simulink library "motdrv_lib"  (Simulink 7.5)
settings: Solver=ode45  StartTime=0.0  StopTime=10.0  RelTol=1e-3
settings Model: Creator=dauger  LastModifiedBy=dauger

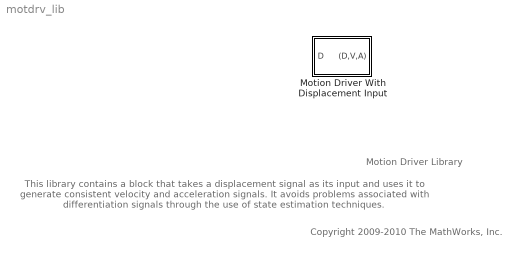
== system motdrv_lib ==
  note: Motion Driver Library
  note: This library contains a block that takes a displacement signal as its input and
      | uses it to generate consistent velocity and acceleration signals.  It avoids problems
      | associated with differentiation signals through the use of state estimation techniques.
  note: Copyright 2009-2010 The MathWorks, Inc.
  Motion Driver With Displacement Input : Subsystem  mask(Motion Driver with Acceleration Input){InitialDisplacement=0, InitialVelocity=0, TimeConstant=1}
      mask prompts: InitialDisplacement "Initial Displacement (units):"; InitialVelocity "Initial Velocity (units/s):"; TimeConstant "Time Constant (s):"
      mask help: This block takes as its input an acceleration and produces a three-dimensional output vector containing a displacement, a velocity and the original acceleration. This is useful for driving SimMechanics actuators with motion. To get correct performance, the user needs to specify the initial displacement and velocity signals.
      mask Display:
      | port_label('input', 1, 'D');
      | port_label('output', 1, '(D,V,A)');

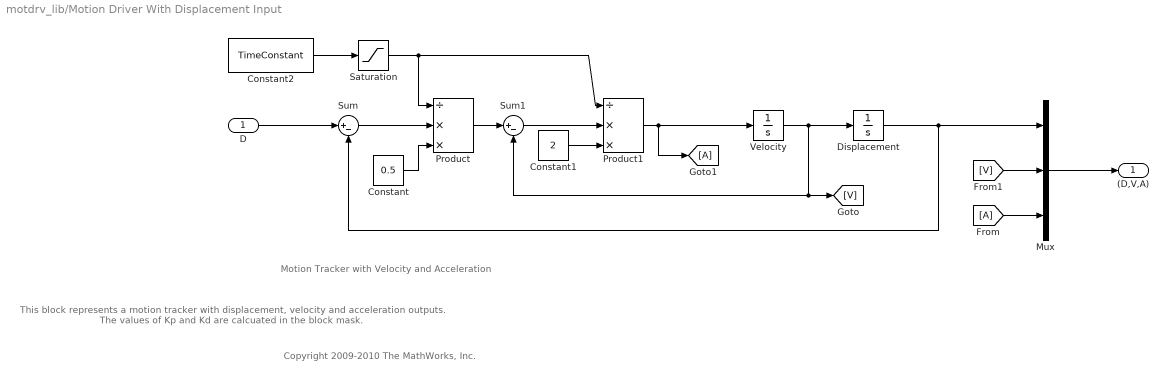
== system motdrv_lib/Motion Driver With Displacement Input ==
  note: Motion Tracker with Velocity and Acceleration
  note: This block represents a motion tracker with displacement, velocity
      | and acceleration outputs.  The values of Kp and Kd are calcuated
      | in the block mask.
  note: Copyright 2009-2010 The MathWorks, Inc.
  D : Inport  PortDimensions=1
  Constant : Constant  Value=0.5  OutDataType=fixdt(1, 16)  OutScaling=2^0
  Constant1 : Constant  Value=2  OutDataType=fixdt(1, 16)  OutScaling=2^0
  Constant2 : Constant  Value=TimeConstant  OutDataType=fixdt(1, 16)  OutScaling=2^0
  Displacement : Integrator  InitialCondition=InitialDisplacement
  Mux : Mux  Inputs=3
  Product : Product  Inputs=/**  OutDataType=fixdt(1, 16)  OutScaling=2^0  RndMeth=Zero
  Product1 : Product  Inputs=/**  OutDataType=fixdt(1, 16)  OutScaling=2^0  RndMeth=Zero
  Saturation : Saturate  UpperLimit=Inf  LowerLimit=eps  OutDataType=fixdt(1, 16)  OutScaling=2^0
      settings: AttributesFormatString=Upper Limit = %<UpperLimit>\nLower Limit = %<LowerLimit>
  Sum : Sum  Inputs=|+-  OutDataType=fixdt(1, 16)  OutScaling=2^0
  Sum1 : Sum  Inputs=|+-  OutDataType=fixdt(1, 16)  OutScaling=2^0
  Velocity : Integrator  InitialCondition=InitialVelocity
  (D,V,A) : Outport  PortDimensions=3
  wires:
  D/1 -> Sum/1
  Sum/1 -> Product/2
  Sum1/1 -> Product1/2
  Mux/1 -> (D,V,A)/1
  Displacement/1 -> Mux/1, Sum/2
  Velocity/1 -> Displacement/1, Sum1/2, [V]
  Product/1 -> Sum1/1
  Product1/1 -> [A], Velocity/1
  Constant/1 -> Product/3
  Constant1/1 -> Product1/3
  Constant2/1 -> Saturation/1
  Saturation/1 -> Product/1, Product1/1
  [V] -> Mux/2
  [A] -> Mux/3
